simulink model "PotholeAlertModel"  (R2025b)
settings: Solver=VariableStepAuto  StartTime=0.0  StopTime=10.0  RelTol=1e-3
values from neighbouring files (symbols this model uses):
  STEERING_THRESHOLD = Simulink.Parameter    [PotholeAlert.m]
libraries: simulink x2
settings Model: Creator=NSA7HC  LastModifiedBy=NSA7HC

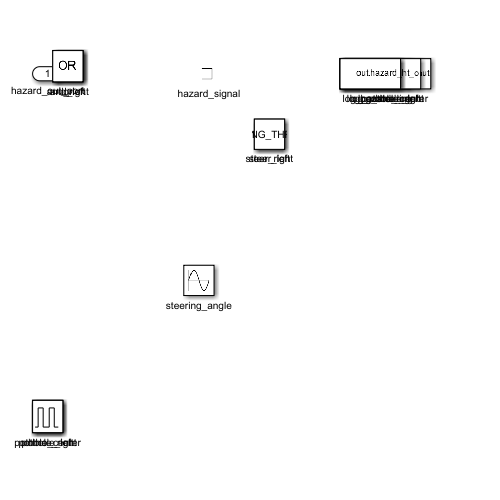
[thumbnail: Simulink's stored preview of the top-level diagram]
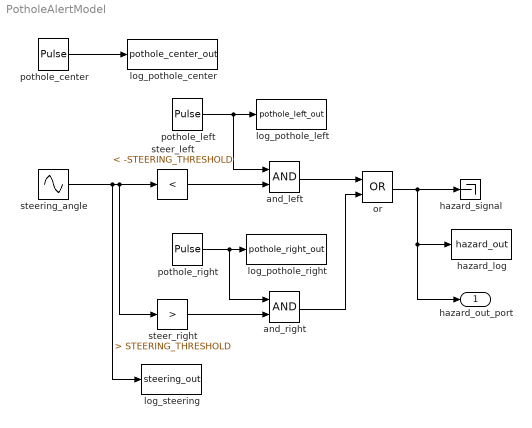
== system PotholeAlertModel ==
  and_left : Logic  AllPortsSameDT=off  OutDataTypeStr=boolean
  and_right : Logic  AllPortsSameDT=off  OutDataTypeStr=boolean
  hazard_log : ToWorkspace  VariableName=hazard_out  SaveFormat=Timeseries  SampleTime=-1
  hazard_signal : Terminator
  log_pothole_center : ToWorkspace  VariableName=pothole_center_out  SaveFormat=Timeseries  SampleTime=-1
  log_pothole_left : ToWorkspace  VariableName=pothole_left_out  SaveFormat=Timeseries  SampleTime=-1
  log_pothole_right : ToWorkspace  VariableName=pothole_right_out  SaveFormat=Timeseries  SampleTime=-1
  log_steering : ToWorkspace  VariableName=steering_out  SaveFormat=Timeseries  SampleTime=-1
  or : Logic  Operator=OR  AllPortsSameDT=off  OutDataTypeStr=boolean
  pothole_center : DiscretePulseGenerator  PulseType=Time based  Period=20  PulseWidth=7.5  PhaseDelay=5.5
  pothole_left : DiscretePulseGenerator  PulseType=Time based  Period=20  PulseWidth=10  PhaseDelay=8.5
  pothole_right : DiscretePulseGenerator  PulseType=Time based  Period=20  PulseWidth=10  PhaseDelay=2
  steer_left : simulink/Logic and Bit Operations/Compare To Constant  relop=<  const=-STEERING_THRESHOLD  OutDataTypeStr=boolean
  steer_right : simulink/Logic and Bit Operations/Compare To Constant  relop=>  const=STEERING_THRESHOLD  OutDataTypeStr=boolean
  steering_angle : Sin  Amplitude=25  Frequency=0.5  SampleTime=0
  hazard_out_port : Outport
  wires:
  pothole_center/1 -> log_pothole_center/1
  pothole_right/1 -> log_pothole_right/1, and_right/1
  and_left/1 -> or/1
  steering_angle/1 -> steer_left/1, steer_right/1, log_steering/1
  steer_left/1 -> and_left/2
  pothole_left/1 -> and_left/1, log_pothole_left/1
  steer_right/1 -> and_right/2
  and_right/1 -> or/2
  or/1 -> hazard_out_port/1, hazard_log/1, hazard_signal/1
